simulink model "processor"  (R2025a)
settings: Solver=VariableStepAuto  StartTime=0.0  StopTime=10.0  RelTol=1e-3
libraries: simulink x9
settings Model: Creator=moham  LastModifiedBy=moham

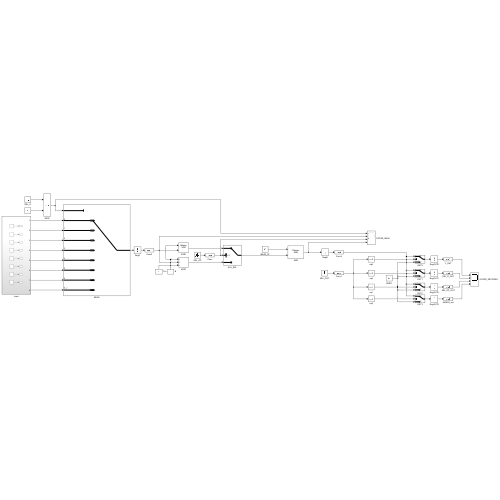
[thumbnail: Simulink's stored preview of the top-level diagram]
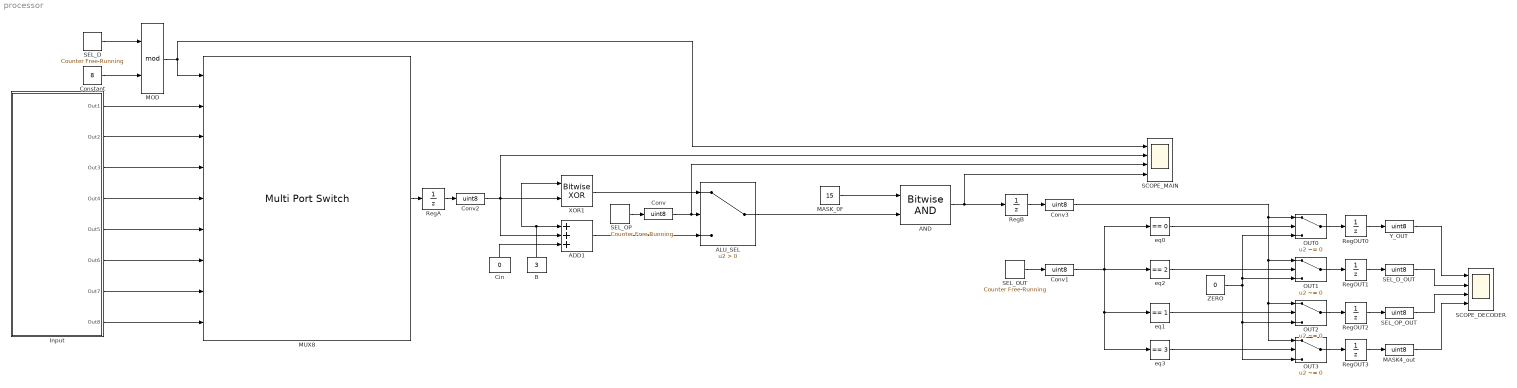
== system processor ==
  ADD1 : Sum  Inputs=+++  OutDataTypeStr=uint8
  ALU_SEL : Switch  Criteria=u2 > Threshold  SaturateOnIntegerOverflow=off  InputSameDT=off
  AND : simulink/Logic and Bit Operations/Bitwise Operator  logicop=AND  UseBitMask=off  NumInputPorts=2  BitMask=bin2dec('11011001')  BitMaskRealWorld=Stored Integer
  B : Constant  Value=3  OutDataTypeStr=uint8
  Cin : Constant  Value=0  OutDataTypeStr=uint8
  Constant : Constant  Value=8  OutDataTypeStr=uint8
  Conv{,1..3} (4 alike) : DataTypeConversion  OutDataTypeStr=uint8  SaturateOnIntegerOverflow=off  RndMeth=Floor
  Input : Subsystem
  MASK4_out : DataTypeConversion  OutDataTypeStr=uint8  SaturateOnIntegerOverflow=off  RndMeth=Floor
  MASK_0F : Constant  Value=15  OutDataTypeStr=uint8
  MOD : Math  Operator=mod
  MUX8 : MultiPortSwitch  DataPortOrder=Zero-based contiguous  Inputs=8  zeroidx=on  SaturateOnIntegerOverflow=off  InputSameDT=off
  OUT{0..3} (4 alike) : Switch  Criteria=u2 ~= 0  SaturateOnIntegerOverflow=off  InputSameDT=off
  RegA : UnitDelay  SampleTime=-1  HasFrameUpgradeWarning=on
  RegB : UnitDelay  SampleTime=-1  HasFrameUpgradeWarning=on
  RegOUT{0..3} (4 alike) : UnitDelay  SampleTime=-1  HasFrameUpgradeWarning=on
  SCOPE_DECODER : Scope  NumInputPorts=4
      settings: ActiveDisplayYMinimum=-9.3903374867629257  ActiveDisplayYMaximum=18.691651705446446
  SCOPE_MAIN : Scope  NumInputPorts=4
      settings: ActiveDisplayYMinimum=-5.1630760998712475  ActiveDisplayYMaximum=11.292715778572749  DataLoggingVariableName=ScopeData3
  SEL_D : simulink/Sources/Counter Free-Running  NumBits=8  tsamp=-1
  SEL_D_OUT : DataTypeConversion  OutDataTypeStr=uint8  SaturateOnIntegerOverflow=off  RndMeth=Floor
  SEL_OP : simulink/Sources/Counter Free-Running  NumBits=2  tsamp=-1
  SEL_OP_OUT : DataTypeConversion  OutDataTypeStr=uint8  SaturateOnIntegerOverflow=off  RndMeth=Floor
  SEL_OUT : simulink/Sources/Counter Free-Running  NumBits=4  tsamp=-1
  XOR1 : simulink/Logic and Bit Operations/Bitwise Operator  logicop=XOR  UseBitMask=off  NumInputPorts=2  BitMask=bin2dec('11011001')  BitMaskRealWorld=Stored Integer
  Y_OUT : DataTypeConversion  OutDataTypeStr=uint8  SaturateOnIntegerOverflow=off  RndMeth=Floor
  ZERO : Constant  Value=0  OutDataTypeStr=uint8
  eq0 : simulink/Logic and Bit Operations/Compare To Constant  relop===  const=0  OutDataTypeStr=boolean
  eq1 : simulink/Logic and Bit Operations/Compare To Constant  relop===  const=1  OutDataTypeStr=boolean
  eq2 : simulink/Logic and Bit Operations/Compare To Constant  relop===  const=2  OutDataTypeStr=boolean
  eq3 : simulink/Logic and Bit Operations/Compare To Constant  relop===  const=3  OutDataTypeStr=boolean
  wires:
  SEL_D/1 -> MOD/1
  Input/1(Out1) -> MUX8/2
  Input/2(Out2) -> MUX8/3
  Input/3(Out3) -> MUX8/4
  Input/4(Out4) -> MUX8/5
  Input/5(Out5) -> MUX8/6
  Input/6(Out6) -> MUX8/7
  Input/7(Out7) -> MUX8/8
  Input/8(Out8) -> MUX8/9
  Cin/1 -> ADD1/3
  B/1 -> XOR1/1, ADD1/1
  MUX8/1 -> RegA/1
  XOR1/1 -> ALU_SEL/1
  ADD1/1 -> ALU_SEL/3
  ALU_SEL/1 -> AND/2
  MASK_0F/1 -> AND/1
  SEL_OP/1 -> Conv/1
  AND/1 -> RegB/1, SCOPE_MAIN/4
  Conv/1 -> SCOPE_MAIN/3, ALU_SEL/2
  MOD/1 -> SCOPE_MAIN/1, MUX8/1
  Constant/1 -> MOD/2
  SEL_OUT/1 -> Conv1/1
  eq0/1 -> OUT0/2
  eq3/1 -> OUT3/2
  OUT0/1 -> RegOUT0/1
  OUT3/1 -> RegOUT3/1
  OUT2/1 -> RegOUT2/1
  OUT1/1 -> RegOUT1/1
  ZERO/1 -> OUT1/3, OUT0/3, OUT2/3, OUT3/3
  eq2/1 -> OUT1/2
  eq1/1 -> OUT2/2
  Conv1/1 -> eq3/1, eq1/1, eq2/1, eq0/1
  RegA/1 -> Conv2/1
  Conv2/1 -> SCOPE_MAIN/2, XOR1/2, ADD1/2
  RegB/1 -> Conv3/1
  Conv3/1 -> OUT2/1, OUT3/1, OUT1/1, OUT0/1
  RegOUT0/1 -> Y_OUT/1
  Y_OUT/1 -> SCOPE_DECODER/1
  RegOUT1/1 -> SEL_D_OUT/1
  SEL_D_OUT/1 -> SCOPE_DECODER/2
  RegOUT2/1 -> SEL_OP_OUT/1
  SEL_OP_OUT/1 -> SCOPE_DECODER/3
  RegOUT3/1 -> MASK4_out/1
  MASK4_out/1 -> SCOPE_DECODER/4

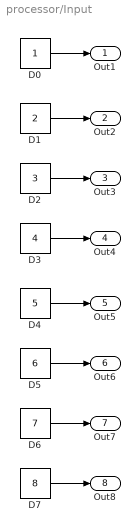
== system processor/Input ==
  D0 : Constant  OutDataTypeStr=uint8
  D1 : Constant  Value=2  OutDataTypeStr=uint8
  D2 : Constant  Value=3  OutDataTypeStr=uint8
  D3 : Constant  Value=4  OutDataTypeStr=uint8
  D4 : Constant  Value=5  OutDataTypeStr=uint8
  D5 : Constant  Value=6  OutDataTypeStr=uint8
  D6 : Constant  Value=7  OutDataTypeStr=uint8
  D7 : Constant  Value=8  OutDataTypeStr=uint8
  Out1 : Outport
  Out2 : Outport  Port=2
  Out3 : Outport  Port=3
  Out4 : Outport  Port=4
  Out5 : Outport  Port=5
  Out6 : Outport  Port=6
  Out7 : Outport  Port=7
  Out8 : Outport  Port=8
  wires:
  D3/1 -> Out4/1
  D2/1 -> Out3/1
  D6/1 -> Out7/1
  D5/1 -> Out6/1
  D4/1 -> Out5/1
  D1/1 -> Out2/1
  D0/1 -> Out1/1
  D7/1 -> Out8/1
